simulink model "Comparison_Systems_Hybrid"  (R2022a)
settings: Solver=ode4  StartTime=0.0  StopTime=0.1  FixedStep=Tsim  RelTol=1e-3
values from neighbouring files (symbols this model uses):
  a = 23.09    [Stetup_HIL.m]
  K = 1    [Stetup_HIL.m]
  T = 1/Fs    (= 0.0025)    [Stetup_HIL.m]
  zg = K*(1-exp(-a*T))    [Stetup_HIL.m]
  zp = exp(-a*T)    [Stetup_HIL.m]
settings Model: Creator=tac29  LastModifiedBy=jayantdubey
settings SolverCC: AlgebraicLoopSolver=TrustRegion
settings DataIOCC: ReturnWorkspaceOutputs=off
settings DebuggingCC: UnconnectedInputMsg=warning  UnconnectedOutputMsg=warning  UnconnectedLineMsg=warning  SFMachineParentedDataDiag=warning  ArithmeticOperatorsInVariantConditions=warning
settings SFSimCC: SimUseLocalCustomCode=off  CustomCodeUndefinedFunction=UseInterfaceOnly
settings RTWCC: RTWUseLocalCustomCode=off  DLArmComputeVersion=19.05
settings CodeAppCC: StateflowObjectComments=on

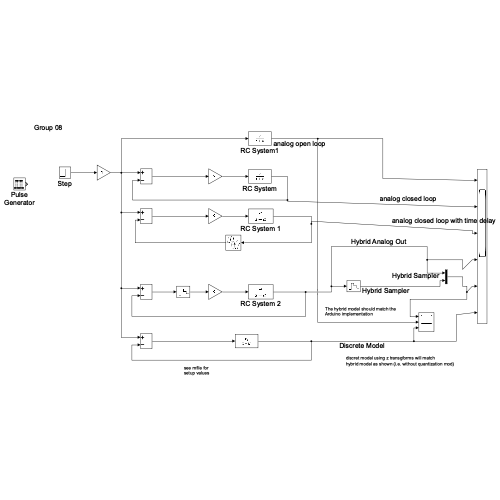
[thumbnail: Simulink's stored preview of the top-level diagram]
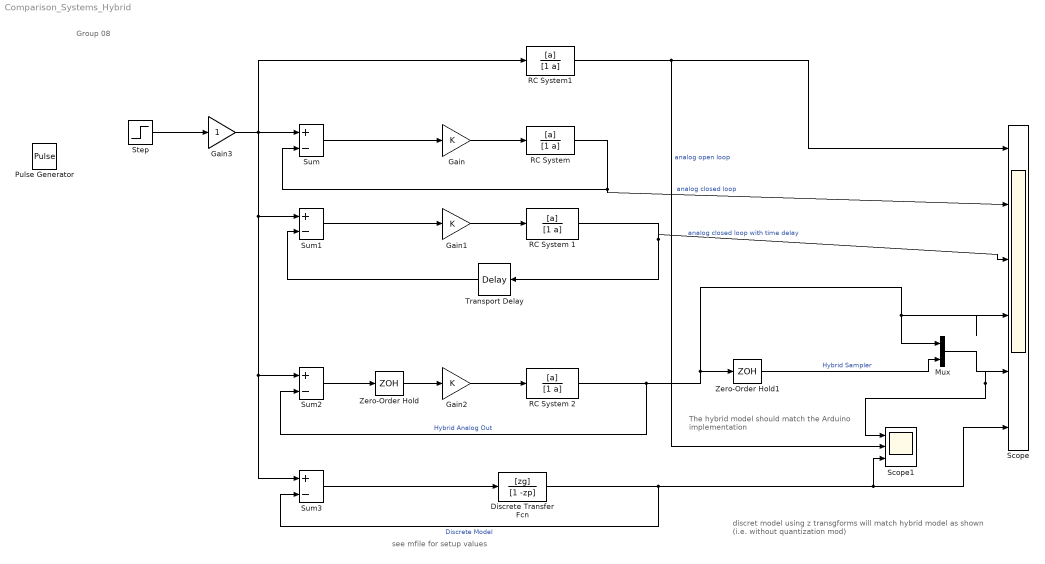
== system Comparison_Systems_Hybrid ==
  note: see mfile for
      | setup values
  note: The hybrid model should match the
      | Arduino implementation
  note: discret model using z transgforms will match
      | hybrid model as shown (i.e. without quantization mod)
  note: Group 08
  Discrete Transfer Fcn : DiscreteTransferFcn  Numerator=[zg]  Denominator=[1 -zp]  SampleTime=T
  Gain : Gain  Gain=K
  Gain1 : Gain  Gain=K
  Gain2 : Gain  Gain=K
  Gain3 : Gain
  Mux : Mux  Inputs=2
  Pulse Generator : DiscretePulseGenerator  Amplitude=10  Period=1000  PulseWidth=10
  RC System : TransferFcn  Numerator=[a]  Denominator=[1 a]
  RC System 1 : TransferFcn  Numerator=[a]  Denominator=[1 a]
  RC System 2 : TransferFcn  Numerator=[a]  Denominator=[1 a]
  RC System1 : TransferFcn  Numerator=[a]  Denominator=[1 a]
  Scope : Scope  NumInputPorts=6
  Scope1 : Scope  NumInputPorts=3
  Step : Step  Time=.01  SampleTime=0
  Sum{,1..3} (4 alike) : Sum  Inputs=+-
  Transport Delay : TransportDelay  DelayTime=T
  Zero-Order Hold : ZeroOrderHold  SampleTime=T
  Zero-Order Hold1 : ZeroOrderHold  SampleTime=T
  wires:
  RC System/1 -> Sum/2, Scope/2  "analog closed loop"
  Sum/1 -> Gain/1
  Gain/1 -> RC System/1
  Sum1/1 -> Gain1/1
  Gain1/1 -> RC System 1/1
  RC System 1/1 -> Transport Delay/1, Scope/3  "analog closed loop with time delay"
  Transport Delay/1 -> Sum1/2
  RC System 2/1 -> Sum2/2, Scope/4, Mux/1, Zero-Order Hold1/1  "Hybrid Analog Out"
  Gain2/1 -> RC System 2/1
  Zero-Order Hold/1 -> Gain2/1
  Sum3/1 -> Discrete Transfer Fcn/1
  Discrete Transfer Fcn/1 -> Sum3/2, Scope/6, Scope1/3  "Discrete Model"
  Gain3/1 -> RC System1/1, Sum3/1, Sum2/1, Sum1/1, Sum/1
  Mux/1 -> Scope1/1, Scope/5
  Zero-Order Hold1/1 -> Mux/2  "Hybrid Sampler"
  Sum2/1 -> Zero-Order Hold/1
  RC System1/1 -> Scope/1, Scope1/2  "analog open loop"
  Step/1 -> Gain3/1
